simulink model "que3"  (R2016a)
settings: Solver=VariableStepAuto  StartTime=0.0  StopTime=10.0  RelTol=1e-3
undefined symbols (not defined in the file): A, B, C, K2, L, x0
settings Model: Creator=X1  LastModifiedBy=X1

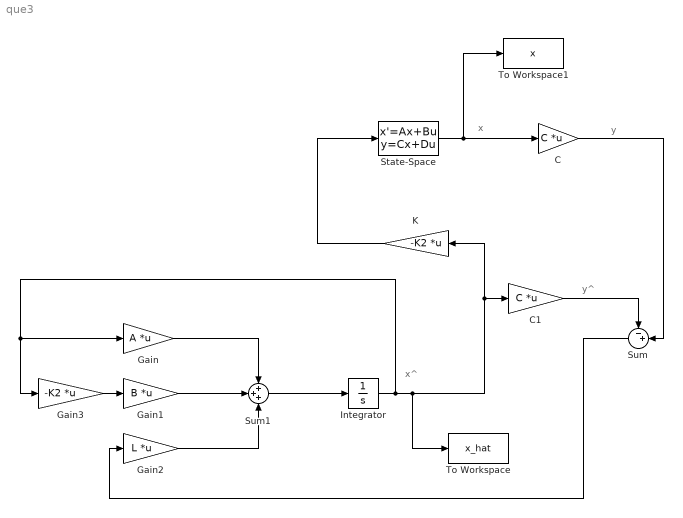
== system que3 ==
  note: y^
  note: x^
  note: x
  note: y
  C : Gain  Gain=C  Multiplication=Matrix(K*u)
  C1 : Gain  Gain=C  Multiplication=Matrix(K*u)
  Gain : Gain  Gain=A  Multiplication=Matrix(K*u)
  Gain1 : Gain  Gain=B  Multiplication=Matrix(K*u)
  Gain2 : Gain  Gain=L  Multiplication=Matrix(K*u)
  Gain3 : Gain  Gain=-K2  Multiplication=Matrix(K*u)
  Integrator : Integrator  InitialCondition=[0 0 0 0 0 0]
  K : Gain  Gain=-K2  Multiplication=Matrix(K*u)
  State-Space : StateSpace  A=A  B=B  C=eye(6)  D=zeros(6,2)  X0=x0
  Sum : Sum  Inputs=-+|
  Sum1 : Sum  Inputs=+++
  To Workspace : ToWorkspace  VariableName=x_hat  SaveFormat=Timeseries  SampleTime=-1
  To Workspace1 : ToWorkspace  VariableName=x  SaveFormat=Timeseries  SampleTime=-1
  wires:
  State-Space/1 -> To Workspace1/1, C/1
  K/1 -> State-Space/1
  Integrator/1 -> To Workspace/1, C1/1, K/1, Gain/1, Gain3/1
  Sum1/1 -> Integrator/1
  Gain1/1 -> Sum1/2
  Gain/1 -> Sum1/1
  Gain2/1 -> Sum1/3
  Gain3/1 -> Gain1/1
  C1/1 -> Sum/1
  Sum/1 -> Gain2/1
  C/1 -> Sum/2
